simulink library "rov_design_analysis"  (Simulink 6.0)
settings: Solver=ode45  SolverMode=SingleTasking  StartTime=0.0  StopTime=10.0  RelTol=1e-3
undefined symbols (not defined in the file or in its folder): amp, At, B, Bt, Ct, cycles, D, den, DL, Do, DQ, DQL, freq, frtest, I, L, m, M, Ma, magnitude, MaU, Mt, nmiss, num, phase, rg, sigbuilder_block, slcm, T, W, xb, xg, Xudot, yb, yg, Yvdot, zb, zg, Zwdot
libraries: simulink_extras x32, simulink x27, rov_design_analysis x15, marine_gnc x10, dspmtrx2 x6, dspstat3 x4
(part 3 of 9)

== system rov_design_analysis/ROV Controller /P-Decoupled  Single loop Controller - 6 DoF  ==
  1. Nonlinear RRC ROV- unperturbed (6DoF) : rov_design_analysis/ROV Models/1. Nonlinear RRC ROV- unperturbed (6DoF)
  Body-fixed to Earth_fixed Transformation1 : Subsystem  AncestorBlock=|
      | rov_design_analysis/ROV Controller
      | Design
      | Applications/2. Passivity-based 
      | and 
      | sliding mode control/Body-fixed to
      | Earth_fixed
      | Transformation3
      mask Display: disp('Euler \nTransformation\n (Transpose)')
  Body-fixed to Earth_fixed Transformation3 : Subsystem  AncestorBlock=|
      | rov_design_analysis/ROV Controller
      | Design
      | Applications/4. Lyapunov PID/Body-fixed to
      | Earth_fixed
      | Transformation1
      mask Display: disp('Euler \nTransformation\n (Transpose)')
  Clock : Clock
      settings: Decimation=10
  Derivative : Derivative
  Euler Transformation 6 DoF : rov_design_analysis/Utilities/Euler Transformation 6 DoF
  Integrator2 : Integrator  Orientation=left
  Model Info : simulink/Model-Wide Utilities/Model Info  InitialBlockCM=None  BlockCM=None  Frame=on  DisplayStringWithTags=|  HorizontalTextAlignment=Center  LeftAlignmentValue=0.5  SourceBlockDiagram=rov_design_analysis  TagMaxNumber=20
      | Passivity-based and Sliding Mode Controller
      | %<Creator>Author
      | %<LastModificationDate>
  Product : Product  Orientation=left  SaturateOnIntegerOverflow=on  RndMeth=Zero  InputSameDT=on
  Product1 : Product  Orientation=left  SaturateOnIntegerOverflow=on  RndMeth=Zero  InputSameDT=on
  Pseudo Inverse (n X n) : Subsystem  AncestorBlock=|  mask(Insert Pseudo Inverse Matrix (for non-square system)){invT=0}
      | rov_design_analysis/Propeller
      | Model/Pseudo Inverse
      | (n X n)
      mask prompts: invT "Insert matrix"
      mask help:
      | Calculate pseudo inverse of  T
      |
      | invT=pinv(T)
      mask Display: disp('Thrust Optim \n (Pseudo-Inverse)')
  Saturation : Saturate  UpperLimit=52.72  LowerLimit=-32.89
  Sign : Signum  Orientation=left
  Subsystem2 : Subsystem
      mask Description: Thruster transfer function
      mask Display: disp('GT')
  Sum1 : Sum  SaturateOnIntegerOverflow=on  InputSameDT=on
  Sum2 : Sum  Inputs=|-+  SaturateOnIntegerOverflow=on  InputSameDT=on
  Sum3 : Sum  Inputs=---  SaturateOnIntegerOverflow=on  InputSameDT=on
  Thruster Matrix : Gain  Gain=T  Multiplication=Matrix(K*u)  SaturateOnIntegerOverflow=on
  Transpose : dspmtrx2/Transpose  Orientation=left  Asize=6  Hermitian=off
  kd : Subsystem
  "kp " : Subsystem
  output body vel : ToWorkspace  VariableName=bout  SampleTime=1  SaveFormat=Array
  output earth pos : ToWorkspace  VariableName=eout  SampleTime=1  SaveFormat=Array
  pipe tracking profile  (Manual) : Subsystem  AncestorBlock=|
      | rov_design_analysis/Scope/pipe tracking
      | profile 
      | (Manual)
  time : ToWorkspace  VariableName=t  SampleTime=1  SaveFormat=Array
  wires:
  Clock/1 -> time/1
  Sum3/1 -> Sum1/2
  Thruster Matrix/1 -> Sum1/1
  Sum1/1 -> 1. Nonlinear RRC ROV- unperturbed (6DoF)/1
  1. Nonlinear RRC ROV- unperturbed (6DoF)/1 -> output body vel/1, Euler Transformation 6 DoF/1, Product/2, Sign/1
  Subsystem2/1("Output ") -> Saturation/1
  pipe tracking profile  (Manual)/1(manual) -> Sum2/1
  Pseudo Inverse (n X n)/1(Out1) -> Subsystem2/1("Input ")
  Saturation/1 -> Thruster Matrix/1
  Integrator2/1 -> Product1/2
  Body-fixed to Earth_fixed Transformation1/1(Output body velocities) -> Pseudo Inverse (n X n)/1(In1)
  Body-fixed to Earth_fixed Transformation3/1(Output body velocities) -> "kp "/1(body vel)
  Product1/1 -> Sum3/3
  Sign/1 -> Product1/1, Transpose/1
  Transpose/1 -> Product/1
  Product/1 -> Integrator2/1
  Sum2/1 -> Body-fixed to Earth_fixed Transformation3/1(Input earth Velocity), Derivative/1
  Derivative/1 -> kd/1(body vel)
  Euler Transformation 6 DoF/1 -> output earth pos/1, Body-fixed to Earth_fixed Transformation1/1(Input earth Velocity), Sum2/2, 1. Nonlinear RRC ROV- unperturbed (6DoF)/2
  kd/1(kd) -> Sum3/2
  "kp "/1(kp) -> Sum3/1

== system rov_design_analysis/ROV Controller /PID  -  4 DoF ==
  PID : Inport  Port=1  LatchInput=off
  Demux1 : Demux
  Mux2 : Mux
  PID Controller1 : simulink_extras/Additional Linear/PID Controller  P=11  I=0  D=1
  PID Controller2 : simulink_extras/Additional Linear/PID Controller  P=11  I=0  D=1
  PID Controller3 : simulink_extras/Additional Linear/PID Controller  P=1  I=0  D=1
  PID Controller4 : simulink_extras/Additional Linear/PID Controller  P=1  I=0  D=1
  " " : Outport
  wires:
  Mux2/1 -> " "/1
  PID/1 -> Demux1/1
  PID Controller4/1 -> Mux2/4
  PID Controller3/1 -> Mux2/3
  PID Controller2/1 -> Mux2/2
  PID Controller1/1 -> Mux2/1
  Demux1/4 -> PID Controller4/1
  Demux1/3 -> PID Controller3/1
  Demux1/2 -> PID Controller2/1
  Demux1/1 -> PID Controller1/1

== system rov_design_analysis/ROV Controller /PID  - 6 DoF ==
  PID : Inport  Port=1  LatchInput=off
  Demux1 : Demux  Outputs=6
  Mux2 : Mux  Inputs=6
  PID Controller1 : simulink_extras/Additional Linear/PID Controller  P=11  I=0  D=1
  PID Controller2 : simulink_extras/Additional Linear/PID Controller  P=11  I=0  D=1
  PID Controller{3..6} (4 alike) : simulink_extras/Additional Linear/PID Controller  P=1  I=0  D=1
  " " : Outport
  wires:
  Demux1/1 -> PID Controller1/1
  Demux1/2 -> PID Controller2/1
  Demux1/3 -> PID Controller3/1
  Demux1/4 -> PID Controller4/1
  PID Controller1/1 -> Mux2/1
  PID Controller2/1 -> Mux2/2
  PID Controller3/1 -> Mux2/3
  PID Controller4/1 -> Mux2/4
  PID/1 -> Demux1/1
  Mux2/1 -> " "/1
  Demux1/5 -> PID Controller5/1
  Demux1/6 -> PID Controller6/1
  PID Controller5/1 -> Mux2/5
  PID Controller6/1 -> Mux2/6

== system rov_design_analysis/ROV Controller /ROV design  in earth fixed frame  PID - 6 DoF ==
  3 to 6 DOF1 : marine_gnc/Models/ Kinetics /Support/3 to 6 DOF
  6 to 3 DOF : Selector  Elements=[1 2 6]  InputPortWidth=6
  "6 to 3 DOF  " : Selector  Orientation=left  Elements=[1 2 6]  InputPortWidth=6
  Constant : Constant  Value=3
  Constant1 : Constant  Value=4
  DP controller1 : marine_gnc/Control/Dynamic  Positioning /DP controller  Kp=diag([0.044e10 0.0069e10 6.9241e10])*0.1*0.1  Kd=diag([0.044e10 0.0069e10 6.9241e10])*2*0.1  Ki=diag([0.044e10 0.0069e10 6.9241e10])*(0.1^3)/10
  Degrees to Radians : simulink_extras/Transformations/Degrees to Radians
  Demux : Demux  Outputs=2
  Model Info : Subsystem  LoadFcn=slcm LoadBlock;  InitFcn=slcm('UpdateAllCMBlocksInThisModelInit')  mask(CMBlock){InitialSaveTempField=, InitialBlockCM=None, BlockCM=None, Frame=on, SaveTempField=, DisplayStringWithTags=|, MaskDisplayString=DP system for a semi-submersible\nexposed for currents. \nAuthor: Thor I. Fossen\n27-Mar-2008 08:24:59, HorizontalTextAlignment=Left, LeftAlignmentValue=0.02, SourceBlockDiagram=rov_design_analysis, TagMaxNumber=20, CMTag1=, CMTag2=, CMTag3=, CMTag4=, CMTag5=, CMTag6=, CMTag7=, CMTag8=, CMTag9=, CMTag10=, CMTag11=, CMTag12=, CMTag13=, CMTag14=, CMTag15=, CMTag16=, CMTag17=, CMTag18=, CMTag19=, CMTag20=}
      mask DisplayStringWithTags=|
      | DP system for a semi-submersible
      | exposed for currents.
      | %<Creator>Author: Thor I. Fossen
      | %<LastModificationDate>
      mask help: This block allows revision control information to be displayed within the model.
      settings: CopyFcn=slcm CopyBlock;  DeleteFcn=slcm Cancel;  PostSaveFcn=slcm('UpdateAllCMBlocksInThisModel')  NameChangeFcn=slcm Rename;  OpenFcn=slcm
      mask Display: text(str2num(LeftAlignmentValue), 0.5, MaskDisplayString, 'HorizontalAlignment', HorizontalTextAlignment)
  Mux : Mux  Inputs=3
  Mux4 : Mux  Inputs=2
  Radians to Degrees : simulink_extras/Transformations/Radians to Degrees
  Selector : Selector  Elements=[1 2]  InputPortWidth=6
  Semi-sub1 : marine_gnc/Examples/Vessels/Semi-sub  D=D  G=G  MA=MA  MRB=MRB
  Step : Step  Time=30  After=10  SampleTime=0
  Transfer Fcn1 : TransferFcn  Denominator=[500 1]
  Transfer Fcn2 : TransferFcn  Denominator=[100 1]
  Transfer Fcn3 : TransferFcn  Denominator=[500 1]
  XY Graph : simulink/Sinks/XY Graph  xmin=-5  xmax=5  ymin=-5  ymax=5  st=-1
  current velocity : Constant  Value=[0.5 0.5 0 0 0 0]
  psi : Fcn  Expr=u(6)
  "psi  " : Scope
      settings: TimeRange=1000  YMin=-2  YMax=10  SaveName=ScopeData3
  wires:
  Constant/1 -> Transfer Fcn1/1  "xd"
  Step/1 -> Transfer Fcn2/1  "psid"
  Degrees to Radians/1 -> Mux/3, Mux4/1
  Constant1/1 -> Transfer Fcn3/1  "yd"
  Demux/1 -> XY Graph/1
  Demux/2 -> XY Graph/2
  Mux/1 -> DP controller1/1
  Transfer Fcn2/1 -> Degrees to Radians/1
  Semi-sub1/1 -> psi/1, Selector/1, "6 to 3 DOF  "/1
  Radians to Degrees/1 -> "psi  "/1
  Mux4/1 -> Radians to Degrees/1
  DP controller1/1 -> 3 to 6 DOF1/1
  psi/1 -> Mux4/2
  Selector/1 -> Demux/1
  current velocity/1 -> Semi-sub1/2
  3 to 6 DOF1/1 -> Semi-sub1/1
  6 to 3 DOF/1 -> DP controller1/3
  "6 to 3 DOF  "/1 -> DP controller1/2
  Semi-sub1/2 -> 6 to 3 DOF/1
  Transfer Fcn1/1 -> Mux/1
  Transfer Fcn3/1 -> Mux/2

== system rov_design_analysis/Thruster  Controller/1. Propeller thrust control - one DoF ==
  Model Info : simulink/Model-Wide Utilities/Model Info  InitialBlockCM=None  BlockCM=None  Frame=on  DisplayStringWithTags=|  HorizontalTextAlignment=Center  LeftAlignmentValue=0.5  SourceBlockDiagram=rov_design_analysis  TagMaxNumber=20
      | Propeller Shaft Speed Control
      | %<Creator>Author: C.S. Chin
      | %<LastModificationDate>
  Qa : Scope
      settings: SaveName=ScopeData4
  Speed control : Subsystem
  Ta : Scope
      settings: TimeRange=60  SaveName=ScopeData5
  Tref : Constant  Value=10
  wires:
  Tref/1 -> Speed control/1(Tref)
  Speed control/1(Ta) -> Ta/1
  Speed control/2(Qa) -> Qa/1

== system rov_design_analysis/Thruster  Controller/2. Thruster Allocation- RRC ROV ==
  vel  (6 DoF) : Inport  Port=1  LatchInput=off
  " input" : Constant  Value=[ 1 1 1 1]'
  Model Info : rov_design_analysis/ROV Models/1. Nonlinear RRC ROV- unperturbed (6DoF)/Model Info  InitialBlockCM=None  BlockCM=None  Frame=on  DisplayStringWithTags=|  HorizontalTextAlignment=Left  LeftAlignmentValue=0.02  SourceBlockDiagram=rov_design_analysis  TagMaxNumber=20
      | Reference:\n
      | [1] C. S. Chin, M. W. S. Lau, E. Low, G. G. Seet.\n Software for Modelling and Simulation of a Remotely Operated Vehicle,\n International Journal of Simulation Modelling, Vol.5, No. 3, p114-125, \n Sept 2006.\n
      | %<Creator>Author: C.S. Chin
      | %<LastModificationDate>
  Selector : Selector  Elements=[1 2 3 6]  InputPortWidth=6
  "thruster allocation " : Subsystem
  volt (4 DoF) : Outport
  wires:
  vel  (6 DoF)/1 -> Selector/1
  Selector/1 -> "thruster allocation "/1(vel)
  " input"/1 -> "thruster allocation "/2(on/off)
  "thruster allocation "/1(volt) -> volt (4 DoF)/1

== system rov_design_analysis/Utilities/6 DoF comparison ==
  eout1 : Inport  Port=1  LatchInput=off
  eout2 : Inport  Port=2  LatchInput=off
  6DOF comparison : Scope  NumInputPorts=6
      settings: TimeRange=200  YMin=-0.2~-0.15~-0.5~-0.2~-0.02~-0.015  YMax=0.3~0.175~0.5~0.2~0.02~0.0175  MaxDataPoints=20000
  Demux1 : Demux  Outputs=6
  Demux2 : Demux  Outputs=6
  Mux{,1..5} (6 alike) : Mux  Inputs=2
  wires:
  Mux5/1 -> 6DOF comparison/6  "yaw"
  Mux4/1 -> 6DOF comparison/5  "pitch"
  Mux3/1 -> 6DOF comparison/4  "roll"
  Mux2/1 -> 6DOF comparison/3  "heave"
  Mux1/1 -> 6DOF comparison/2  "sway"
  Mux/1 -> 6DOF comparison/1  "surge"
  eout2/1 -> Demux1/1
  eout1/1 -> Demux2/1
  Demux1/6 -> Mux5/2
  Demux1/5 -> Mux4/2
  Demux1/4 -> Mux3/2
  Demux1/3 -> Mux2/2
  Demux1/2 -> Mux1/2
  Demux2/6 -> Mux5/1  "yaw"
  Demux2/5 -> Mux4/1  "pitch"
  Demux2/4 -> Mux3/1  "roll"
  Demux2/3 -> Mux2/1  "heave"
  Demux2/2 -> Mux1/1  "sway"
  Demux1/1 -> Mux/2  "surge"
  Demux2/1 -> Mux/1  "surge"

== system rov_design_analysis/Utilities/6 to 4 DoF ==
  6 DOF : Inport  Port=1  LatchInput=off
  Kt1 : Gain  Gain=0.0013  SaturateOnIntegerOverflow=on
  Selector : Selector  Elements=[1 2 3 6]  InputPortWidth=6
  square1 : Math  Operator=square  SaturateOnIntegerOverflow=on
  4DOF : Outport
  wires:
  Selector/1 -> 4DOF/1
  6 DOF/1 -> Selector/1
  square1/1 -> Kt1/1

== system rov_design_analysis/Utilities/6 to 4 or 2 DoF ==
  6 DOF : Inport  Port=1  LatchInput=off
  Kt1 : Gain  Gain=0.0013  SaturateOnIntegerOverflow=on
  Selector : Selector  Elements=[1 2 3 6]  InputPortWidth=6
  Selector1 : Selector  Elements=[ 4 5 ]  InputPortWidth=6
  square1 : Math  Operator=square  SaturateOnIntegerOverflow=on
  4DOF : Outport
  2 DOF : Outport  Port=2
  wires:
  Selector1/1 -> 2 DOF/1
  Selector/1 -> 4DOF/1
  6 DOF/1 -> Selector/1, Selector1/1
  square1/1 -> Kt1/1

== system rov_design_analysis/Utilities/Body Velocity Scope (6 DoF)   ==
  In : Inport  Port=1  LatchInput=off
  Demux : Demux  Outputs=6
  p : Scope
      settings: TickLabels=on  YMin=-0.125  YMax=0.2  DataFormat=Array
  q : Scope
      settings: TickLabels=on  TimeRange=200  YMin=-0.05  YMax=0.15  DataFormat=Array
  r : Scope
      settings: TickLabels=on  TimeRange=200  YMin=-0.05  YMax=0.15  DataFormat=Array
  u : Scope
      settings: TickLabels=on  TimeRange=50  YMin=-0.025  YMax=0.375  DataFormat=Array
  v : Scope
      settings: TickLabels=on  YMin=-0.02  YMax=0.1  DataFormat=Array
  w : Scope
      settings: TickLabels=on  TimeRange=50  YMin=-0.0025  YMax=0.0375  DataFormat=Array
  wires:
  Demux/1 -> u/1
  Demux/2 -> v/1
  Demux/3 -> w/1
  In/1 -> Demux/1
  Demux/4 -> p/1
  Demux/5 -> q/1
  Demux/6 -> r/1

== system rov_design_analysis/Utilities/Earth Position  Scope (6 DoF)  ==
  In : Inport  Port=1  LatchInput=off
  Demux1 : Demux  Outputs=6
  pitch : Scope
      settings: TickLabels=on  YMin=-0.05  YMax=0.15  DataFormat=Array
  roll : Scope
      settings: TickLabels=on  YMin=-0.125  YMax=0.2  DataFormat=Array
  x : Scope
      settings: TickLabels=on  TimeRange=50  YMin=0  YMax=0.375  DataFormat=Array
  y : Scope
      settings: TickLabels=on  YMin=-0.15  YMax=0.175  DataFormat=Array
  yaw : Scope
      settings: TickLabels=on  YMin=0  YMax=1.75  DataFormat=Array
  z : Scope
      settings: TickLabels=on  TimeRange=50  YMin=-0.0025  YMax=0.0375  DataFormat=Array
  wires:
  In/1 -> Demux1/1
  Demux1/1 -> x/1
  Demux1/6 -> yaw/1
  Demux1/5 -> pitch/1
  Demux1/4 -> roll/1
  Demux1/3 -> z/1
  Demux1/2 -> y/1

== system rov_design_analysis/Utilities/Euler Transformation 4 DoF   ==
  yaw angle : Inport  Port=1  LatchInput=off
  vel : Inport  Port=2  LatchInput=off
  (zg.W - zb.B)cY.sX : Fcn  Expr=cos(u[1])-sin(u[1])
  (zg.W - zb.B)cY.sX1 : Fcn  Expr=sin(u[1])+cos(u[1])
  Constant : Constant
  Constant1 : Constant
  Constant2 : Constant  Value=0
  Intregrator2 : Integrator
  Mux1 : Mux  Inputs=6
  Product : Product  RndMeth=Zero
  eout : Outport  InitialOutput=0
  wires:
  (zg.W - zb.B)cY.sX/1 -> Mux1/1
  yaw angle/1 -> (zg.W - zb.B)cY.sX/1, (zg.W - zb.B)cY.sX1/1
  (zg.W - zb.B)cY.sX1/1 -> Mux1/2
  Mux1/1 -> Product/1
  vel/1 -> Product/2
  Product/1 -> Intregrator2/1
  Intregrator2/1 -> eout/1
  Constant1/1 -> Mux1/6
  Constant/1 -> Mux1/5
  Constant2/1 -> Mux1/3, Mux1/4

== system rov_design_analysis/Utilities/Euler Transformation 6 DoF ==
  vel : Inport  Port=1  LatchInput=off
  Demux : Demux  Outputs=2
  Demux1 : Demux  Outputs=2
  Intregrator2 : Integrator
  Mux1 : Mux  Inputs=2
  Terminator : Terminator
  Transformation matrix R : Subsystem
      mask Display: disp('Transformation R')
  Transformation matrix T : Subsystem
      mask Display: disp('Transformation T')
  eout : Outport  InitialOutput=0
  wires:
  Demux1/1 -> Terminator/1
  Transformation matrix T/1(translational earth velocity) -> Mux1/1
  Transformation matrix R/1(angular earth velocity) -> Mux1/2
  Demux1/2 -> Transformation matrix R/2(angular position), Transformation matrix T/2(angular position)
  vel/1 -> Demux/1
  Demux/1 -> Transformation matrix T/1(translational body velocity)
  Demux/2 -> Transformation matrix R/1(angular body  velocity)
  Intregrator2/1 -> Demux1/1, eout/1
  Mux1/1 -> Intregrator2/1

== system rov_design_analysis/Utilities/Inverse Euler Transformation 4 DoF ==
  yaw angle : Inport  Port=1  LatchInput=off
  (zg.W - zb.B)cY.sX : Fcn  Expr=cos(u[1])+sin(u[1])
  (zg.W - zb.B)cY.sX1 : Fcn  Expr=-sin(u[1])+cos(u[1])
  Constant : Constant
  Constant1 : Constant
  Constant2 : Constant  Value=0
  Mux1 : Mux  Inputs=6
  out : Outport
  wires:
  (zg.W - zb.B)cY.sX/1 -> Mux1/1
  (zg.W - zb.B)cY.sX1/1 -> Mux1/2
  yaw angle/1 -> (zg.W - zb.B)cY.sX1/1, (zg.W - zb.B)cY.sX/1
  Constant1/1 -> Mux1/6
  Constant/1 -> Mux1/5
  Constant2/1 -> Mux1/3, Mux1/4
  Mux1/1 -> out/1  "J_inv"

== system rov_design_analysis/Utilities/Joystrick (4 DoF) ==
  Gain : Gain  Gain=0.5
  Integrator : Integrator
  Subsystem : Subsystem  mask{dzlow=10, dzhigh=3, slowdown=on}
      mask prompts: dzlow "Deadzone lower limit"; dzhigh "Deadzone upper limit"; slowdown "real speed"
      mask help:
      | Enter deadzone Settings in percent of stick movement.
      | Slow down simulation to real world speed by checking box.
  Surge velocity (m/s) : Display
  Sway Velocity (m/s) : Display
  Terminator : Terminator
  Terminator1 : Terminator
  Terminator2 : Terminator
  Yaw (rad) : Display
  heave velocity (m/s) : Display
  yaw2 : Display
  u : Outport
  v : Outport  Port=2
  w : Outport  Port=3
  yaw : Outport  Port=4
  wires:
  Subsystem/1(LX) -> Sway Velocity (m/s)/1, v/1
  Subsystem/2(LY) -> Surge velocity (m/s)/1, u/1
  Subsystem/3(RX) -> Terminator1/1
  Subsystem/4(RY) -> yaw2/1, Integrator/1
  Subsystem/5(RT) -> Gain/1
  Subsystem/6(LT) -> Terminator/1
  Subsystem/7(buttons) -> Terminator2/1
  Gain/1 -> heave velocity (m/s)/1, w/1
  Integrator/1 -> Yaw (rad)/1, yaw/1

== system rov_design_analysis/Utilities/Modes indicator-hort/vert/station - 6 DoF ==
  inputs : Inport  Port=1  LatchInput=off
  1 : Subsystem
      mask Display: disp('surge')
  2 : Subsystem  AncestorBlock=|
      | rov_design_analysis/Scope
      | Utilities/thust  allocation
      | (manual)/1
      mask Display: disp('sway')
  3 : Subsystem  AncestorBlock=|
      | rov_design_analysis/Scope
      | Utilities/thust  allocation
      | (manual)/1
      mask Display: disp('heave')
  4 : Subsystem  AncestorBlock=|
      | rov_design_analysis/Scope
      | Utilities/thust  allocation
      | (manual)/1
      mask Display: disp('roll')
  5 : Subsystem  AncestorBlock=|
      | rov_design_analysis/Scope
      | Utilities/thust  allocation
      | (manual)/1
      mask Display: disp('pitch')
  6 : Subsystem  AncestorBlock=|
      | rov_design_analysis/Scope
      | Utilities/thust  allocation
      | (manual)/1
      mask Display: disp('yaw')
  Constant : Constant
  Constant1 : Constant  Value=2
  Constant2 : Constant  Value=3
  Demux : Demux  Outputs=6
  Demux1 : Demux  Outputs=6
  Mux : Mux  Inputs=6
  Mux1 : Mux  Inputs=3
  Product : Product  OutDataTypeMode=double  SaturateOnIntegerOverflow=on  RndMeth=Zero
  Product1 : Product  OutDataTypeMode=double  SaturateOnIntegerOverflow=on  RndMeth=Zero
  Product2 : Product  OutDataTypeMode=double  SaturateOnIntegerOverflow=on  RndMeth=Zero
  horizontal  plane : Logic  Inputs=3  AllPortsSameDT=off
  station keeping : Logic  Inputs=4  AllPortsSameDT=off
  vertical  plane : Logic  Inputs=3  AllPortsSameDT=off
  eout : Outport
  hort/vert/station : Outport  Port=2
  wires:
  Demux/1 -> 1/1(In)
  1/1(Out) -> Mux/1
  2/1(Out1) -> Mux/2
  3/1(Out1) -> Mux/3
  Demux/2 -> 2/1(In1)
  4/1(Out1) -> Mux/4
  5/1(Out1) -> Mux/5
  6/1(Out1) -> Mux/6
  inputs/1 -> Demux/1
  horizontal  plane/1 -> Product/2
  Constant/1 -> Product/1
  vertical  plane/1 -> Product1/2
  Constant1/1 -> Product1/1
  station keeping/1 -> Product2/2
  Constant2/1 -> Product2/1
  Product/1 -> Mux1/1
  Product1/1 -> Mux1/2
  Product2/1 -> Mux1/3
  Mux1/1 -> hort/vert/station/1
  Demux/3 -> 3/1(In1)
  Demux/4 -> 4/1(In1)
  Demux/5 -> 5/1(In1)
  Demux/6 -> 6/1(In1)
  Mux/1 -> Demux1/1, eout/1
  Demux1/1 -> horizontal  plane/1, vertical  plane/1, station keeping/1
  Demux1/2 -> horizontal  plane/2, station keeping/2
  Demux1/6 -> horizontal  plane/3, station keeping/4
  Demux1/3 -> vertical  plane/2
  Demux1/5 -> vertical  plane/3
  Demux1/4 -> station keeping/3

== system rov_design_analysis/Utilities/Process Capability  (1 DoF) ==
  mean : Inport  Port=1  LatchInput=off
  desired : Inport  Port=2  LatchInput=off
  std : Inport  Port=3  LatchInput=off
  "Gain  " : Gain  Gain=3
  Mean  1 : dspstat3/Mean  DialogController=dspDDGCreate  DialogControllerArgs=DataTag0  run=off  reset_popup=None  roundingMode=Floor  overflowMode=off
  Standard Deviation1 : dspstat3/Standard Deviation  run=off  reset_popup=None
  "cpk " : Subsystem
  cpk : Outport
  wires:
  std/1 -> Standard Deviation1/1
  "cpk "/1(cpk) -> cpk/1
  desired/1 -> "cpk "/2(desired)
  mean/1 -> Mean  1/1
  "Gain  "/1 -> "cpk "/3(3*sigma)
  Standard Deviation1/1 -> "Gain  "/1
  Mean  1/1 -> "cpk "/1(mean)

== system rov_design_analysis/Utilities/Switching sequence ==
  Add2 : Sum  Inputs=+++++++  OutScaling=2^-10
  Signal Builder2 : Subsystem  Tag=STV Subsys  LoadFcn=sigbuilder_block('load');  StartFcn=sigbuilder_block('start');  StopFcn=sigbuilder_block('stop');  ClipboardFcn=sigbuilder_block('clipboard');  mask(Sigbuilder block){}
      mask help: Sigbuilder GUI
      mask init:
      | if ~strcmp(get_param(bdroot(gcbh),'SimulationStatus'),'stopped') tuvar = sigbuilder_block('maskInit'); end
      settings: CopyFcn=sigbuilder_block('copy');  DeleteFcn=sigbuilder_block('delete');  ModelCloseFcn=sigbuilder_block('modelClose');  PreSaveFcn=sigbuilder_block('preSave');  NameChangeFcn=sigbuilder_block('namechange');  OpenFcn=sigbuilder_block('open',[0 19.5 768 499.5 ]);  CloseFcn=sigbuilder_block('close');
      mask Display: plot(0,0,100,100,[10,10,40,40,10],[80,20,20,80,80],[40,10],[50,50], [40,27,10],[65,72,56],[40,25,25,10],[28,28,43,43]);
  " " : Outport
  wires:
  Signal Builder2/1(Signal 1) -> Add2/1
  Signal Builder2/2(Signal 2) -> Add2/2
  Signal Builder2/3(Signal 3) -> Add2/3
  Signal Builder2/4(Signal 4) -> Add2/4
  Signal Builder2/5(Signal 5) -> Add2/5
  Signal Builder2/6(Signal 6) -> Add2/6
  Signal Builder2/7(Signal 7) -> Add2/7
  Add2/1 -> " "/1

== system rov_design_analysis/Utilities/Switching sequence - Controller ==
  t : Inport  Port=1  LatchInput=off
  Constant1 : Constant  Value=t3
  Constant10 : Constant  Value=t5
  Constant11 : Constant  Value=6
  Constant2 : Constant
  Constant4 : Constant  Value=2
  Constant5 : Constant  Value=4
  Constant6 : Constant  Value=t2
  Constant7 : Constant  Value=3
  Constant8 : Constant  Value=5
  Constant9 : Constant  Value=t4
  Relational Operator{1..5} (5 alike) : RelationalOperator  LogicOutDataTypeMode=Boolean
  Switch{,1..4} (5 alike) : Switch
  t1 : Constant  Value=t1
  Out-sequence : Outport
  wires:
  t/1 -> Relational Operator2/1, Relational Operator3/1, Relational Operator1/1, Relational Operator4/1, Relational Operator5/1
  t1/1 -> Relational Operator2/2
  Constant4/1 -> Switch/1
  Relational Operator2/1 -> Switch/2
  Constant2/1 -> Switch/3
  Switch/1 -> Switch1/3
  Constant6/1 -> Relational Operator3/2
  Constant7/1 -> Switch1/1
  Relational Operator3/1 -> Switch1/2
  Switch1/1 -> Switch2/3
  Constant5/1 -> Switch2/1
  Constant1/1 -> Relational Operator1/2
  Relational Operator1/1 -> Switch2/2
  Switch2/1 -> Switch3/3
  Constant8/1 -> Switch3/1
  Constant9/1 -> Relational Operator4/2
  Relational Operator4/1 -> Switch3/2
  Switch3/1 -> Switch4/3
  Constant10/1 -> Relational Operator5/2
  Relational Operator5/1 -> Switch4/2
  Constant11/1 -> Switch4/1
  Switch4/1 -> Out-sequence/1

== system rov_design_analysis/Utilities/Time capture ==
  Clock1 : Clock
      settings: Decimation=10
  time : ToWorkspace  VariableName=t  SampleTime=1  SaveFormat=Array
  wires:
  Clock1/1 -> time/1

== system rov_design_analysis/Utilities/Unit Conversion ==
  in : Inport  Port=1  LatchInput=off
  Gain : Gain  Gain=k  SaturateOnIntegerOverflow=on
  out : Outport
  wires:
  Gain/1 -> out/1
  in/1 -> Gain/1

== system rov_design_analysis/Utilities/Z-score (1 DoF) ==
  mean : Inport  Port=1  LatchInput=off
  desired : Inport  Port=2  LatchInput=off
  std : Inport  Port=3  LatchInput=off
  "Gain  " : Gain  Gain=3
  Mean  1 : dspstat3/Mean  DialogController=dspDDGCreate  DialogControllerArgs=DataTag3  run=off  reset_popup=None  roundingMode=Floor  overflowMode=off
  Standard Deviation1 : dspstat3/Standard Deviation  run=off  reset_popup=None
  "Zscore " : Subsystem
  Zscore : Outport
  wires:
  Mean  1/1 -> "Zscore "/1(mean)
  Standard Deviation1/1 -> "Gain  "/1
  "Gain  "/1 -> "Zscore "/3(3*sigma)
  mean/1 -> Mean  1/1
  desired/1 -> "Zscore "/2(desired)
  "Zscore "/1(Zscore) -> Zscore/1
  std/1 -> Standard Deviation1/1

== system rov_design_analysis/Utilities/pipe tracking profile  (4 DoF) ==
  Mux : Mux
  x : Step  Time=0  After=0  SampleTime=0
  y : Step  Time=0  After=0  SampleTime=0
  yaw : Step  Time=0  After=-1.57  SampleTime=0
  z : Step  Time=0  After=-50  SampleTime=0
  4 DOF inputs : Outport
  wires:
  yaw/1 -> Mux/4
  x/1 -> Mux/1
  y/1 -> Mux/2
  z/1 -> Mux/3
  Mux/1 -> 4 DOF inputs/1

== system rov_design_analysis/Utilities/pipe tracking profile  (6 DoF) ==
  Mux : Mux  Inputs=6
  pitch : Step  Time=0  After=-50  SampleTime=0
  roll : Step  Time=0  After=0  SampleTime=0
  x : Step  Time=0  After=0  SampleTime=0
  y : Step  Time=0  After=0  SampleTime=0
  yaw : Step  Time=0  After=-1.57  SampleTime=0
  z : Step  Time=0  After=-50  SampleTime=0
  6DOF inputs : Outport
  wires:
  Mux/1 -> 6DOF inputs/1
  z/1 -> Mux/3
  y/1 -> Mux/2
  x/1 -> Mux/1
  yaw/1 -> Mux/6
  roll/1 -> Mux/4
  pitch/1 -> Mux/5

== system rov_design_analysis/Utilities/pipeline  tracking planner  (6 DoF)  ==
  select : Inport  Port=1  LatchInput=off
  Multiport Switch : MultiPortSwitch  Inputs=2
  coupled input : Subsystem
  manual : Constant  Value="[20 0  0   0  0  1.57]'"  OutDataTypeMode=double
  output body vel9 : ToWorkspace  VariableName=plane  SampleTime=1  SaveFormat=Structure With Time
  switching input sequence : Subsystem
  pipe-6DOFs : Outport
  wires:
  switching input sequence/1(" ") -> output body vel9/1, coupled input/1(In)
  Multiport Switch/1 -> pipe-6DOFs/1
  select/1 -> Multiport Switch/1
  manual/1 -> Multiport Switch/3
  coupled input/1(Out) -> Multiport Switch/2

== system rov_design_analysis/Analysis/Model Info/EmptySubsystem ==

== system rov_design_analysis/Identification/Frequency Response Analysis/1.open ==

== system rov_design_analysis/Identification/Frequency Response Analysis/2.Plot Bode ==

== system rov_design_analysis/Identification/Frequency Response Analysis/3. Plot Mag ==

== system rov_design_analysis/Identification/Frequency Response Analysis/Correlation Frquency Analyzer ==
  note: Simulink implementation of a correlation frequency response analyser
  Sine wave : Inport  Port=1  LatchInput=off
  in : Inport  Port=2  LatchInput=off
  "Averaging 1/T " : Gain  Gain=frtest/((cycles-nmiss)*pi)  SaturateOnIntegerOverflow=on
  Clock : Clock
  CoSine Wave : Sin  Frequency=frtest  Phase=pi/2  SampleTime=0
  Complex to Magnitude-Angle : ComplexToMagnitudeAngle
  Gain : Gain  Gain=20  SaturateOnIntegerOverflow=on
  Imaginary : Integrator
  Math Function : Math  Operator=log10  SaturateOnIntegerOverflow=on
  Product : Product  SaturateOnIntegerOverflow=on  RndMeth=Zero  InputSameDT=on
  Product1 : Product  SaturateOnIntegerOverflow=on  RndMeth=Zero  InputSameDT=on
  Radians to Degrees : simulink_extras/Transformations/Radians to Degrees
  Real-Imag to Complex : RealImagToComplex
  Scope : Scope
      settings: TimeRange=60  YMin=0  YMax=0.08
  Switch to start the integration after the transient has died down : Switch  Threshold=2*nmiss*pi/frtest  SaturateOnIntegerOverflow=on  InputSameDT=on
  real : Integrator
  zero : Constant  Value=0
  mag : Outport
  deg : Outport  Port=2
  wires:
  Product1/1 -> Imaginary/1
  CoSine Wave/1 -> Product1/2
  Product/1 -> real/1
  Switch to start the integration after the transient has died down/1 -> "Averaging 1/T "/1
  "Averaging 1/T "/1 -> Product/1, Product1/1, Scope/1
  real/1 -> Real-Imag to Complex/1
  Imaginary/1 -> Real-Imag to Complex/2
  Real-Imag to Complex/1 -> Complex to Magnitude-Angle/1
  Math Function/1 -> Gain/1
  Complex to Magnitude-Angle/2 -> Radians to Degrees/1
  Complex to Magnitude-Angle/1 -> Math Function/1
  in/1 -> Switch to start the integration after the transient has died down/1
  zero/1 -> Switch to start the integration after the transient has died down/3
  Clock/1 -> Switch to start the integration after the transient has died down/2
  Gain/1 -> mag/1
  Radians to Degrees/1 -> deg/1
  Sine wave/1 -> Product/2

== system rov_design_analysis/Identification/Frequency Response Analysis/Model Info1 ==
  EmptySubsystem : Subsystem

== system rov_design_analysis/Identification/Frequency Response Analysis/System under test ==
  In1 : Inport  Port=1  LatchInput=off
  Transfer Fcn : TransferFcn  Numerator=num  Denominator=den
  Out1 : Outport
  wires:
  In1/1 -> Transfer Fcn/1
  Transfer Fcn/1 -> Out1/1

== system rov_design_analysis/Identification/Kalman filter  /0.5*(P+P') ==
  P : Inport  Port=1  LatchInput=off
  "    " : Math  Operator=transpose  SaturateOnIntegerOverflow=on
  Gain6 : Gain  Gain=0.5  SaturateOnIntegerOverflow=on
  Sum12 : Sum  Inputs=|++  SaturateOnIntegerOverflow=on
  P=P' : Outport
  wires:
  P/1 -> Sum12/2, "    "/1  "P"
  "    "/1 -> Sum12/1  "P'"
  Sum12/1 -> Gain6/1
  Gain6/1 -> P=P'/1

== system rov_design_analysis/Identification/Kalman filter  /matrices ==
  A-matrix : Constant  Value="[0 1 0 0 0;  -w_o^2  -2*w_o*lambda 0 0 0; 0 0 0 1 0; 0 0 0 -1/T -K/T; 0 0 0 0 -1/T_b]"
  EQE'-matrix : Constant  Value=[0 0 0 0 0; 0 q1 0 0 0; 0 0 0 0 0; 0 0 0 q2 0; 0 0 0 0 q3]
  A : Outport
  EQE' : Outport  Port=2
  wires:
  A-matrix/1 -> A/1
  EQE'-matrix/1 -> EQE'/1

== system rov_design_analysis/Identification/kalman filter- observer + i/o noise/1. Load RRCROV parameters ==

== system rov_design_analysis/Identification/kalman filter- observer + i/o noise/2. Load thruster & ROV model(in state space & tfm) ==

== system rov_design_analysis/Identification/kalman filter- observer + i/o noise/Double click here to start loading data and mu-syn design ==

== system rov_design_analysis/Propeller Models/1.  propeller with motor characteristics - 1DoF (account for dynamic variation in ua,up)/axial flow dynamic ==
  Ta : Inport  Port=1  LatchInput=off
  vel : Inport  Port=2  LatchInput=off
  (1-w)u : Product  SaturateOnIntegerOverflow=on  RndMeth=Zero  InputSameDT=on
  1/mt : Product  SaturateOnIntegerOverflow=on  RndMeth=Zero  InputSameDT=on
  Ap : Constant  Value=pi*0.1^2/4
  Integratr1 : Integrator
  L : Constant  Value=0.01
  Math Function : Math  Operator=reciprocal  SaturateOnIntegerOverflow=on
  Math Function1 : Math  Operator=reciprocal  SaturateOnIntegerOverflow=on
  Sum : Sum  Inputs=|+--  SaturateOnIntegerOverflow=on  InputSameDT=on
  Sum1 : Sum  Inputs=|+-  SaturateOnIntegerOverflow=on  InputSameDT=on
  Sum2 : Sum  Inputs=|+-  SaturateOnIntegerOverflow=on  InputSameDT=on
  dt : Constant  Value=0.01
  dt*lupl*(up-ua) : Product  Inputs=3  SaturateOnIntegerOverflow=on  RndMeth=Zero  InputSameDT=on
  dt1 : Constant
  dto : Constant  Value=0.05
  dto*up : Product  SaturateOnIntegerOverflow=on  RndMeth=Zero  InputSameDT=on
  gamma : Constant  Value=2
  lupl : Abs  SaturateOnIntegerOverflow=on
  mt : Product  Inputs=4  SaturateOnIntegerOverflow=on  RndMeth=Zero  InputSameDT=on
  mt/0.05 : Product  SaturateOnIntegerOverflow=on  RndMeth=Zero  InputSameDT=on
  mt1 : Product  Inputs=3  SaturateOnIntegerOverflow=on  RndMeth=Zero  InputSameDT=on
  p : Constant  Value=1024
  w : Constant  Value=0.4
  ua : Outport
  wires:
  1/mt/1 -> Integratr1/1
  mt1/1 -> dt*lupl*(up-ua)/2
  Ap/1 -> mt1/1, mt/3
  p/1 -> mt1/2, mt/2
  dt/1 -> mt1/3
  mt/0.05/1 -> dto*up/2
  mt/1 -> mt/0.05/1, Math Function/1
  Math Function1/1 -> mt/0.05/2
  dto/1 -> Math Function1/1
  L/1 -> mt/4
  gamma/1 -> mt/1
  Math Function/1 -> 1/mt/1
  Sum/1 -> 1/mt/2
  vel/1 -> (1-w)u/1
  Ta/1 -> Sum/1
  dt*lupl*(up-ua)/1 -> Sum/3
  w/1 -> Sum2/2
  dt1/1 -> Sum2/1
  Sum2/1 -> (1-w)u/2
  (1-w)u/1 -> Sum1/2
  Sum1/1 -> dt*lupl*(up-ua)/3
  lupl/1 -> dt*lupl*(up-ua)/1
  Integratr1/1 -> ua/1, Sum1/1, lupl/1, dto*up/1
  dto*up/1 -> Sum/2

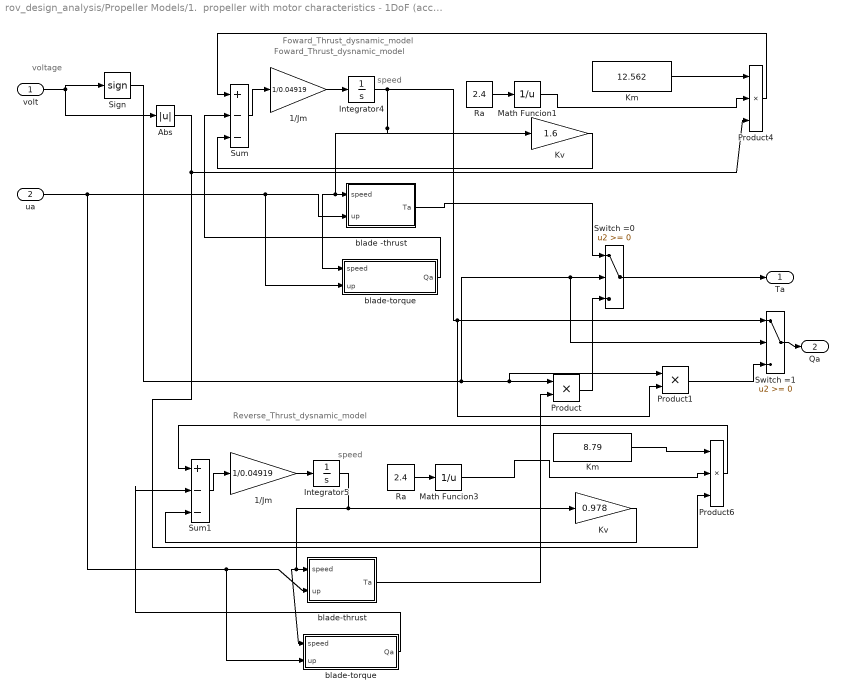
== system rov_design_analysis/Propeller Models/1.  propeller with motor characteristics - 1DoF (account for dynamic variation in ua,up)/motor and propeller dynamic  ==
  note: speed
  note: Reverse_Thrust_dysnamic_model
  note: speed
  note: voltage
  note: Foward_Thrust_dysnamic_model
  note: Foward_Thrust_dysnamic_model
  volt : Inport  Port=1  LatchInput=off
  ua : Inport  Port=2  LatchInput=off
  1/Jm : Gain  Gain=1/0.04919  SaturateOnIntegerOverflow=on
  "1/Jm " : Gain  Gain=1/0.04919  SaturateOnIntegerOverflow=on
  Abs : Abs  SaturateOnIntegerOverflow=on
  Integrator4 : Integrator
  Integrator5 : Integrator
  Km : Constant  Value=12.562
  "Km " : Constant  Value=8.79
  Kv : Gain  Gain=1.6  SaturateOnIntegerOverflow=on
  "Kv " : Gain  Gain=0.978  SaturateOnIntegerOverflow=on
  Math Funcion1 : Math  Operator=reciprocal  SaturateOnIntegerOverflow=on
  Math Funcion3 : Math  Operator=reciprocal  SaturateOnIntegerOverflow=on
  Product : Product  SaturateOnIntegerOverflow=on  RndMeth=Zero  InputSameDT=on
  Product1 : Product  SaturateOnIntegerOverflow=on  RndMeth=Zero  InputSameDT=on
  Product4 : Product  Inputs=3  SaturateOnIntegerOverflow=on  RndMeth=Zero  InputSameDT=on
  Product6 : Product  Inputs=3  SaturateOnIntegerOverflow=on  RndMeth=Zero  InputSameDT=on
  Ra : Constant  Value=2.4
  "Ra " : Constant  Value=2.4
  Sign : Signum
  Sum : Sum  Inputs=|+--  SaturateOnIntegerOverflow=on  InputSameDT=on
  Sum1 : Sum  Inputs=|+--  SaturateOnIntegerOverflow=on  InputSameDT=on
  Switch =0 : Switch  SaturateOnIntegerOverflow=on  InputSameDT=on
  Switch =1 : Switch  SaturateOnIntegerOverflow=on  InputSameDT=on
  blade -thrust : Subsystem
  "blade-thrust " : Subsystem
  blade-torque : Subsystem
  "blade-torque " : Subsystem
  Ta : Outport
  Qa : Outport  Port=2
  wires:
  Switch =1/1 -> Qa/1
  Switch =0/1 -> Ta/1
  Kv/1 -> Sum/3
  Product1/1 -> Switch =1/3
  Integrator4/1 -> Product1/2, Switch =1/1, blade-torque/1(speed), blade -thrust/1(speed), Kv/1
  Integrator5/1 -> "blade-torque "/1(speed), "blade-thrust "/1(speed), "Kv "/1
  ua/1 -> "blade-torque "/2(up), "blade-thrust "/2(up), blade-torque/2(up), blade -thrust/2(up)
  "blade-thrust "/1(Ta) -> Product/2
  "Kv "/1 -> Sum1/3
  Product6/1 -> Sum1/1
  "1/Jm "/1 -> Integrator5/1
  Sum1/1 -> "1/Jm "/1
  "blade-torque "/1(Qa) -> Sum1/2
  "Ra "/1 -> Math Funcion3/1
  Product4/1 -> Sum/1
  Abs/1 -> Product6/3, Product4/3
  blade -thrust/1(Ta) -> Switch =0/1
  1/Jm/1 -> Integrator4/1
  Sum/1 -> 1/Jm/1
  blade-torque/1(Qa) -> Sum/2
  Ra/1 -> Math Funcion1/1
  Sign/1 -> Product1/1, Product/1, Switch =1/2, Switch =0/2
  Product/1 -> Switch =0/3
  volt/1 -> Abs/1, Sign/1
  Km/1 -> Product4/1
  Math Funcion1/1 -> Product4/2
  "Km "/1 -> Product6/1
  Math Funcion3/1 -> Product6/2

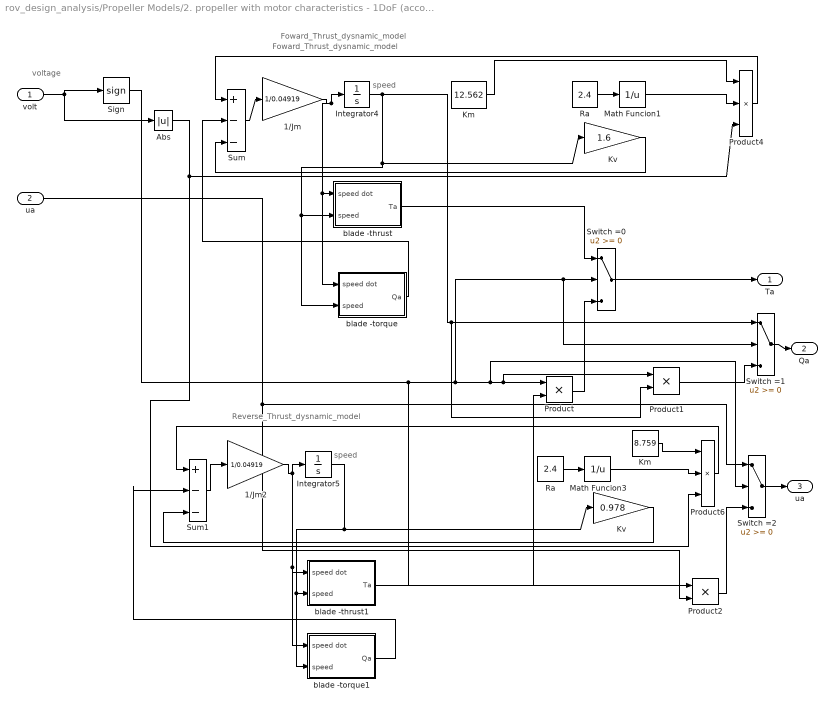
== system rov_design_analysis/Propeller Models/2. propeller with motor characteristics - 1DoF (account for ua only)/motor and propeller dynamic  ==
  note: Foward_Thrust_dysnamic_model
  note: Foward_Thrust_dysnamic_model
  note: voltage
  note: speed
  note: Reverse_Thrust_dysnamic_model
  note: speed
  volt : Inport  Port=1  LatchInput=off
  ua : Inport  Port=2  LatchInput=off
  1/Jm : Gain  Gain=1/0.04919  SaturateOnIntegerOverflow=on
  1/Jm2 : Gain  Gain=1/0.04919  SaturateOnIntegerOverflow=on
  Abs : Abs  SaturateOnIntegerOverflow=on
  Integrator4 : Integrator
  Integrator5 : Integrator
  Km : Constant  Value=12.562
  "Km " : Constant  Value=8.759
  "Kv " : Gain  Gain=1.6  SaturateOnIntegerOverflow=on
  "Kv   " : Gain  Gain=0.978  SaturateOnIntegerOverflow=on
  Math Funcion1 : Math  Operator=reciprocal  SaturateOnIntegerOverflow=on
  Math Funcion3 : Math  Operator=reciprocal  SaturateOnIntegerOverflow=on
  Product : Product  SaturateOnIntegerOverflow=on  RndMeth=Zero  InputSameDT=on
  Product1 : Product  SaturateOnIntegerOverflow=on  RndMeth=Zero  InputSameDT=on
  Product2 : Product  SaturateOnIntegerOverflow=on  RndMeth=Zero  InputSameDT=on
  Product4 : Product  Inputs=3  SaturateOnIntegerOverflow=on  RndMeth=Zero  InputSameDT=on
  Product6 : Product  Inputs=3  SaturateOnIntegerOverflow=on  RndMeth=Zero  InputSameDT=on
  Ra : Constant  Value=2.4
  "Ra " : Constant  Value=2.4
  Sign : Signum
  Sum : Sum  Inputs=|+--  SaturateOnIntegerOverflow=on  InputSameDT=on
  Sum1 : Sum  Inputs=|+--  SaturateOnIntegerOverflow=on  InputSameDT=on
  Switch =0 : Switch  SaturateOnIntegerOverflow=on  InputSameDT=on
  Switch =1 : Switch  SaturateOnIntegerOverflow=on  InputSameDT=on
  Switch =2 : Switch  SaturateOnIntegerOverflow=on  InputSameDT=on
  blade -thrust : Subsystem
  blade -thrust1 : Subsystem  AncestorBlock=|
      | rov_design_analysis/Propeller
      | Model/ propeller with motor
      | characteristics
      | (steady state)/motor and propeller
      | dynamic /blade -thrust
  blade -torque : Subsystem  AncestorBlock=|
      | rov_design_analysis/Propeller
      | Model/ propeller with motor
      | characteristics
      | (steady state)/motor and propeller
      | dynamic /blade -thrust
  blade -torque1 : Subsystem  AncestorBlock=|
      | rov_design_analysis/Propeller
      | Model/ propeller with motor
      | characteristics
      | (steady state)/motor and propeller
      | dynamic /blade -torque
  Ta : Outport
  Qa : Outport  Port=2
  "ua " : Outport  Port=3
  wires:
  volt/1 -> Sign/1, Abs/1
  Product/1 -> Switch =0/3
  Sign/1 -> Switch =0/2, Switch =1/2, Product/1, Product1/1, Switch =2/2, Product2/1
  Ra/1 -> Math Funcion1/1
  Km/1 -> Product4/1
  Math Funcion1/1 -> Product4/2
  blade -torque/1(Qa) -> Sum/2
  Sum/1 -> 1/Jm/1
  1/Jm/1 -> Integrator4/1, blade -thrust/1(speed dot), blade -torque/1(speed dot)
  blade -thrust/1(Ta) -> Switch =0/1
  Abs/1 -> Product4/3, Product6/3
  Product4/1 -> Sum/1
  "Ra "/1 -> Math Funcion3/1
  blade -torque1/1(Qa) -> Sum1/2
  Sum1/1 -> 1/Jm2/1
  1/Jm2/1 -> Integrator5/1, blade -thrust1/1(speed dot), blade -torque1/1(speed dot)
  Product6/1 -> Sum1/1
  "Kv   "/1 -> Sum1/3
  blade -thrust1/1(Ta) -> Product/2
  Math Funcion3/1 -> Product6/2
  ua/1 -> Switch =2/1, Product2/2
  Integrator5/1 -> blade -thrust1/2(speed), blade -torque1/2(speed), "Kv   "/1
  Integrator4/1 -> Switch =1/1, Product1/2, blade -thrust/2(speed), blade -torque/2(speed), "Kv "/1
  Product1/1 -> Switch =1/3
  Switch =0/1 -> Ta/1
  Switch =1/1 -> Qa/1
  Switch =2/1 -> "ua "/1
  Product2/1 -> Switch =2/3
  "Kv "/1 -> Sum/3
  "Km "/1 -> Product6/1

== system rov_design_analysis/Propeller Models/5. first-order thruster dynamic - 4 DoF/SubSystem11 ==
  volt : Inport  Port=1  LatchInput=off
  Transfer Fcn : TransferFcn  Numerator=0.97  Denominator=[0.02 1]
  thrust : Outport
  wires:
  Transfer Fcn/1 -> thrust/1
  volt/1 -> Transfer Fcn/1

== system rov_design_analysis/Propeller Models/5. first-order thruster dynamic - 4 DoF/SubSystem12 ==
  volt : Inport  Port=1  LatchInput=off
  Transfer Fcn : TransferFcn  Numerator=0.97  Denominator=[0.02 1]
  thrust : Outport
  wires:
  Transfer Fcn/1 -> thrust/1
  volt/1 -> Transfer Fcn/1

== system rov_design_analysis/Propeller Models/5. first-order thruster dynamic - 4 DoF/SubSystem5 ==
  volt : Inport  Port=1  LatchInput=off
  Transfer Fcn : TransferFcn  Numerator=0.97  Denominator=[0.02 1]
  thrust : Outport
  wires:
  Transfer Fcn/1 -> thrust/1
  volt/1 -> Transfer Fcn/1

== system rov_design_analysis/Propeller Models/5. first-order thruster dynamic - 4 DoF/SubSystem6 ==
  volt : Inport  Port=1  LatchInput=off
  Transfer Fcn : TransferFcn  Numerator=0.97  Denominator=[0.02 1]
  thrust : Outport
  wires:
  Transfer Fcn/1 -> thrust/1
  volt/1 -> Transfer Fcn/1

== system rov_design_analysis/Propeller Models/6. first order motor dynamic- 1DoF (no account for ua,up)/first order motor dynamic ==
  volt : Inport  Port=1  LatchInput=off
  1/time const : Constant  Value=0.1
  Integrator : Integrator
  Product : Product  SaturateOnIntegerOverflow=on  RndMeth=Zero  InputSameDT=on
  Sum : Sum  Inputs=|+-  SaturateOnIntegerOverflow=on  InputSameDT=on
  torque : Outport
  wires:
  1/time const/1 -> Product/1
  Product/1 -> Sum/1
  Sum/1 -> Integrator/1
  Integrator/1 -> Sum/2, torque/1
  volt/1 -> Product/2

== system rov_design_analysis/Propeller Models/6. first order motor dynamic- 1DoF (no account for ua,up)/propeller Load Torque ==
  n : Inport  Port=1  LatchInput=off
  Abs : Abs  Orientation=left  SaturateOnIntegerOverflow=on
  Constant4 : Constant  Orientation=left  Value=5
  D : Constant  Orientation=left  Value=0.1
  KQ : Constant  Orientation=left  Value=0.00022
  Math Function1 : Math  Orientation=left  Operator=pow  SaturateOnIntegerOverflow=on
  Product1 : Product  Orientation=left  Inputs=5  SaturateOnIntegerOverflow=on  RndMeth=Zero  InputSameDT=on
  "seawater density " : Constant  Orientation=left  Value=1024
  Qa : Outport
  wires:
  "seawater density "/1 -> Product1/1
  Math Function1/1 -> Product1/2
  KQ/1 -> Product1/3
  Abs/1 -> Product1/4
  n/1 -> Abs/1, Product1/5
  Product1/1 -> Qa/1
  D/1 -> Math Function1/1
  Constant4/1 -> Math Function1/2

== system rov_design_analysis/Propeller Models/6. first order motor dynamic- 1DoF (no account for ua,up)/propeller thruster ==
  n : Inport  Port=1  LatchInput=off
  Abs : Abs  Orientation=left  SaturateOnIntegerOverflow=on
  Constant4 : Constant  Orientation=left  Value=4
  D : Constant  Orientation=left  Value=0.1
  KT : Constant  Orientation=left  Value=0.0022
  Math Function1 : Math  Orientation=left  Operator=pow  SaturateOnIntegerOverflow=on
  Product1 : Product  Orientation=left  Inputs=5  SaturateOnIntegerOverflow=on  RndMeth=Zero  InputSameDT=on
  pw : Constant  Orientation=left  Value=1024
  Ta : Outport
  wires:
  pw/1 -> Product1/1
  Math Function1/1 -> Product1/2
  KT/1 -> Product1/3
  Abs/1 -> Product1/4
  n/1 -> Abs/1, Product1/5
  Product1/1 -> Ta/1
  D/1 -> Math Function1/1
  Constant4/1 -> Math Function1/2

== system rov_design_analysis/Propeller Models/6. first order motor dynamic- 1DoF (no account for ua,up)/propeller Shaft Dynamic ==
  Qm : Inport  Port=1  LatchInput=off
  Qa : Inport  Port=2  LatchInput=off
  2*pi : Constant  Value=2*pi
  Integrator : Integrator
  Km : Gain  Orientation=left  Gain=12.562  SaturateOnIntegerOverflow=on
  Math Function : Math  Operator=reciprocal  SaturateOnIntegerOverflow=on
  Product : Product  Inputs=3  SaturateOnIntegerOverflow=on  RndMeth=Zero  InputSameDT=on
  Sum : Sum  Inputs=|+--  SaturateOnIntegerOverflow=on  InputSameDT=on
  shaft inertia : Constant  Value=0.0492
  n : Outport
  wires:
  2*pi/1 -> Product/1
  Math Function/1 -> Product/2
  shaft inertia/1 -> Math Function/1
  Product/1 -> Integrator/1
  Sum/1 -> Product/3
  Km/1 -> Sum/3
  Integrator/1 -> n/1, Km/1
  Qm/1 -> Sum/1
  Qa/1 -> Sum/2

== system rov_design_analysis/ROV Models/ Linear RRC ROV- unperturbed (6DoF)/More Info ==

== system rov_design_analysis/ROV Models/ ROMEO ROV (6DoF)   / Load   ==

== system rov_design_analysis/ROV Models/ ROMEO ROV (6DoF)   /Centripetal & Coriolis ==
  vel : Inport  Orientation=up  Port=1  LatchInput=off
  Demux : Demux  Orientation=up  Outputs=2
  Mux : Mux  Inputs=2
  Product{1..5} (5 alike) : Product  SaturateOnIntegerOverflow=on  RndMeth=Zero  InputSameDT=on
  Rg : Constant  Value=rg
  Sum : Sum  SaturateOnIntegerOverflow=on  InputSameDT=on
  Sum1 : Sum  SaturateOnIntegerOverflow=on  InputSameDT=on
  inertia(3x3) : Gain  Gain=I*eye(3)+[0 0 0;0 0 0;0 0 0]  Multiplication=Matrix(K*u)  SaturateOnIntegerOverflow=on
  "mass(3x3) " : Gain  Gain=m*eye(3)+[0 0 0;0 0 0;0 0 0]  Multiplication=Matrix(K*u)  SaturateOnIntegerOverflow=on
  "mass(3x3)   " : Gain  Gain=m*eye(3)+[0 0 0;0 0 0;0 0 0]  Multiplication=Matrix(K*u)  SaturateOnIntegerOverflow=on
  force : Outport  InitialOutput=0
  wires:
  Product1/1 -> Sum/2
  "mass(3x3)   "/1 -> Product2/1
  Product2/1 -> Sum/1
  Rg/1 -> Product3/2, "mass(3x3)   "/1
  Product3/1 -> Product4/2
  Product4/1 -> Sum1/1
  Product5/1 -> Product2/2, Sum1/2
  Sum1/1 -> "mass(3x3) "/1
  Demux/2 -> Product5/1, Product3/1, Product4/1, Product1/1, inertia(3x3)/1
  Demux/1 -> Product5/2
  vel/1 -> Demux/1
  inertia(3x3)/1 -> Product1/2
  "mass(3x3) "/1 -> Mux/1
  Sum/1 -> Mux/2
  Mux/1 -> force/1

== system rov_design_analysis/ROV Models/ ROMEO ROV (6DoF)   /Hydrodynamic  Damping1 ==
  vel : Inport  Port=1  LatchInput=off
  D quadratic : Gain  Gain=-diag(DQ)  SaturateOnIntegerOverflow=on
  Product : Product  SaturateOnIntegerOverflow=on  RndMeth=Zero  InputSameDT=on
  |u| : Abs  SaturateOnIntegerOverflow=on
  damping force : Outport  InitialOutput=0
  wires:
  Product/1 -> D quadratic/1
  vel/1 -> Product/1, |u|/1
  |u|/1 -> Product/2
  D quadratic/1 -> damping force/1

== system rov_design_analysis/ROV Models/ ROMEO ROV (6DoF)   /Hydrodynamic  Damping2 ==
  vel : Inport  Port=1  LatchInput=off
  D quadratic : Gain  Gain=0  SaturateOnIntegerOverflow=on
  damping force : Outport  InitialOutput=0
  wires:
  D quadratic/1 -> damping force/1
  vel/1 -> D quadratic/1

== system rov_design_analysis/ROV Models/ ROMEO ROV (6DoF)   /Mass Inertia Matrix ==
  In : Inport  Port=1  LatchInput=off
  inverse M : Gain  Gain=inv(M-Ma)  Multiplication=Matrix(K*u)  SaturateOnIntegerOverflow=on
  Out : Outport
  wires:
  inverse M/1 -> Out/1
  In/1 -> inverse M/1

== system rov_design_analysis/ROV Models/ ROMEO ROV (6DoF)   /Restoring Forces ==
  pos : Inport  Port=1  LatchInput=off
  (xg.W-xb.B)cY.cX : Fcn  Expr=(xg*W - xb*B)*cos(u[2])*cos(u[1])
  (zg.W - zb.B)cY.sX : Fcn  Expr=((zg * W - zb * B) * cos(u[2])) * sin(u[1])
  (zg.W - zb.B)sY : Fcn  Expr=(zg*W - zb*B)*sin(u[2])
  -(xg.W-xb.B)cY.sX : Fcn  Expr=-(xg*W - xb*B)*cos(u[2])*sin(u[1])
  -(yg.W-yb.B)cY.cX : Fcn  Expr=-(yg*W - yb*B)*cos(u[2])*cos(u[1])
  -(yg.W-yb.B)sY : Fcn  Expr=-(yg*W - yb*B)*sin(u[2])
  -cY.cX : Fcn  Expr=-cos(u[2])*cos(u[1])
  -cY.sX : Fcn  Expr=-cos(u[2])*sin(u[1])
  Demux : Demux  Outputs=2
  Gain : Gain  Gain=W-B  SaturateOnIntegerOverflow=on
  Mux : Mux  Inputs=3
  Mux1 : Mux
  Sum : Sum  SaturateOnIntegerOverflow=on  InputSameDT=on
  Sum1 : Sum  SaturateOnIntegerOverflow=on  InputSameDT=on
  Sum2 : Sum  SaturateOnIntegerOverflow=on  InputSameDT=on
  Terminator : Terminator
  sY : Fcn  Expr=sin(u[2])
  gravitational force : Outport  InitialOutput=0
  wires:
  Sum2/1 -> Mux1/4
  -(yg.W-yb.B)sY/1 -> Sum2/1
  -(xg.W-xb.B)cY.sX/1 -> Sum2/2
  Sum1/1 -> Mux1/3
  (xg.W-xb.B)cY.cX/1 -> Sum1/1
  (zg.W - zb.B)sY/1 -> Sum1/2
  Sum/1 -> Mux1/2
  (zg.W - zb.B)cY.sX/1 -> Sum/1
  -(yg.W-yb.B)cY.cX/1 -> Sum/2
  Gain/1 -> Mux1/1
  Mux/1 -> Gain/1
  -cY.cX/1 -> Mux/3
  -cY.sX/1 -> Mux/2
  sY/1 -> Mux/1
  Mux1/1 -> gravitational force/1
  Demux/2 -> -(xg.W-xb.B)cY.sX/1, -(yg.W-yb.B)sY/1, (zg.W - zb.B)sY/1, (xg.W-xb.B)cY.cX/1, -(yg.W-yb.B)cY.cX/1, (zg.W - zb.B)cY.sX/1, sY/1, -cY.sX/1, -cY.cX/1
  Demux/1 -> Terminator/1
  pos/1 -> Demux/1

== system rov_design_analysis/ROV Models/ ROMEO ROV (6DoF)   /pert ==
  In : Inport  Port=1  LatchInput=off
  inp : Inport  Port=2  LatchInput=off
  D linear3 : Gain  Gain=2  SaturateOnIntegerOverflow=on
  Product : Product  RndMeth=Zero
  Sine Wave-pert : Sin  Amplitude=0.1  SampleTime=0
  Sum6 : Sum  Inputs=|++  SaturateOnIntegerOverflow=on  InputSameDT=on
  on/off : Outport
  wires:
  D linear3/1 -> Sum6/1
  Sine Wave-pert/1 -> Product/1
  Product/1 -> Sum6/2
  inp/1 -> Product/2
  In/1 -> D linear3/1
  Sum6/1 -> on/off/1

== system rov_design_analysis/ROV Models/ ROMEO ROV (6DoF)   /pert1 ==
  In : Inport  Port=1  LatchInput=off
  inp : Inport  Port=2  LatchInput=off
  D linear3 : Gain  Gain=2  SaturateOnIntegerOverflow=on
  Product : Product  RndMeth=Zero
  Sine Wave-pert : Sin  Amplitude=0.1  SampleTime=0
  Sum6 : Sum  Inputs=|++  SaturateOnIntegerOverflow=on  InputSameDT=on
  on/off : Outport
  wires:
  D linear3/1 -> Sum6/1
  Sine Wave-pert/1 -> Product/1
  Product/1 -> Sum6/2
  inp/1 -> Product/2
  In/1 -> D linear3/1
  Sum6/1 -> on/off/1

== system rov_design_analysis/ROV Models/ ROMEO ROV (6DoF)   /upper limit (diag) ==
  In : Inport  Port=1  LatchInput=off
  inverse M : Gain  Gain=-diag([21.724-21.1403 51.7013-51.7012 94.3-92.451 4.2176-3.6191 7.1148-2.6427 4.7673-2.3033])  Multiplication=Matrix(K*u)  SaturateOnIntegerOverflow=on
  Out : Outport
  wires:
  inverse M/1 -> Out/1
  In/1 -> inverse M/1
